simulink model "linear_system"  (R2022a)
settings: Solver=ode45  StartTime=0.0  StopTime=10  RelTol=1e-3
values from neighbouring files (symbols this model uses):
  A = [A1 A2; A3 A4]    [params.m]
  B = [B1; B2]    [params.m]
  C = diag([1 1 1 1])    [params.m]
  D = [0; 0; 0; 0]    [params.m]
  K = [1 1 1 1]    [params.m]
settings Model: Creator=epyur  LastModifiedBy=epyur
settings SolverCC: ZeroCrossControl=DisableAll

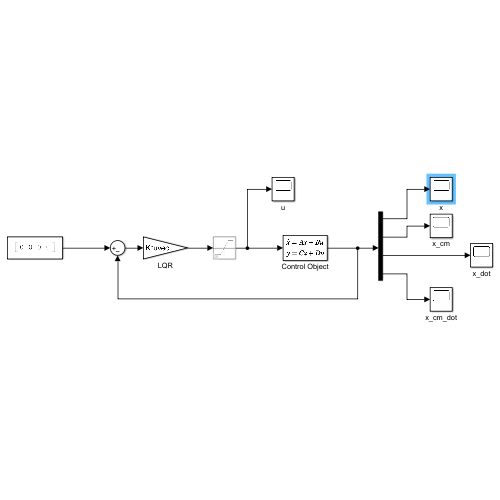
[thumbnail: Simulink's stored preview of the top-level diagram]
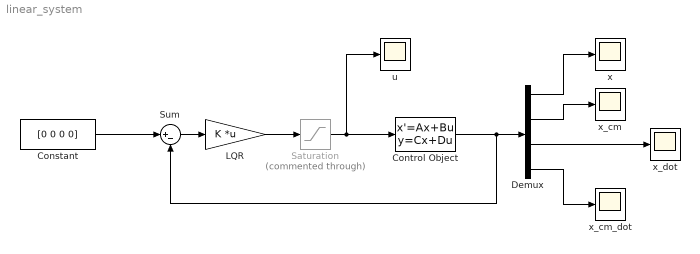
== system linear_system ==
  Constant : Constant  Value=[0 0 0 0]  VectorParams1D=off
  Control Object : StateSpace  A=A  B=B  C=C  D=D  InitialCondition=[0 -0.144 0 0]  ParameterTunability=Unconstrained
  Demux : Demux
  LQR : Gain  Gain=K  Multiplication=Matrix(K*u) (u vector)
  Saturation : Saturate  Commented=through  UpperLimit=24  LowerLimit=-24
  Sum : Sum  Inputs=|+-
  u : Scope
  x : Scope
  x_cm : Scope
  x_cm_dot : Scope
  x_dot : Scope
  wires:
  Sum/1 -> LQR/1
  Constant/1 -> Sum/1
  Control Object/1 -> Sum/2, Demux/1
  Demux/1 -> x/1
  Demux/2 -> x_cm/1
  Demux/3 -> x_dot/1
  Demux/4 -> x_cm_dot/1
  LQR/1 -> Saturation/1
  Saturation/1 -> u/1, Control Object/1
